simulink model "model2_sim"  (R2016a)
settings: Solver=VariableStepAuto  StartTime=0.0  StopTime=30  MaxStep=0.001  RelTol=1e-6
values from neighbouring files (symbols this model uses):
  damp_spring = 0    [model2.m]
  DC_delay = 0.005    [model1.m]    (also in model2.m)
  DC_max_force = 400    [model1.m]    (also in model2.m = 200)
  DC_PID_D = 0    [model1.m]    (also in model2.m = 1000)
  DC_PID_I = 0    [model1.m]    (also in model2.m)
  DC_PID_N = 100    [model2.m]
  DC_PID_P = 0    [model1.m]    (also in model2.m)
  k_cutoffspring = 20000    [model2.m]
  k_spring = 2500    [model2.m]
  linear_act_delay = 0.1    [model1.m]    (also in model2.m)
  linear_act_max = 0.25    [model1.m]    (also in model2.m = 0.5)
  linear_act_speed = 0.1    [model1.m]    (also in model2.m = 0.05)
  m_bed = 10    [model1.m]    (also in model2.m)
  m_payload = m_bed + m_patient    (= 40)    [model1.m]    (also in model2.m)
  max_offset = 0.1    [model1.m]    (also in model2.m)
  noise_rate = 0.1    [model1.m]    (also in model2.m)
  noise_rate_limit = 10    [model2.m]
  noise_start_time = 3    [model1.m]    (also in model2.m)
  patient_sit_pace = 50    [model2.m]
libraries: simulink x5, vrlib x3
settings Model: Creator=Perttu  LastModifiedBy=Perttu
settings SolverCC: InitialStep=0.0005

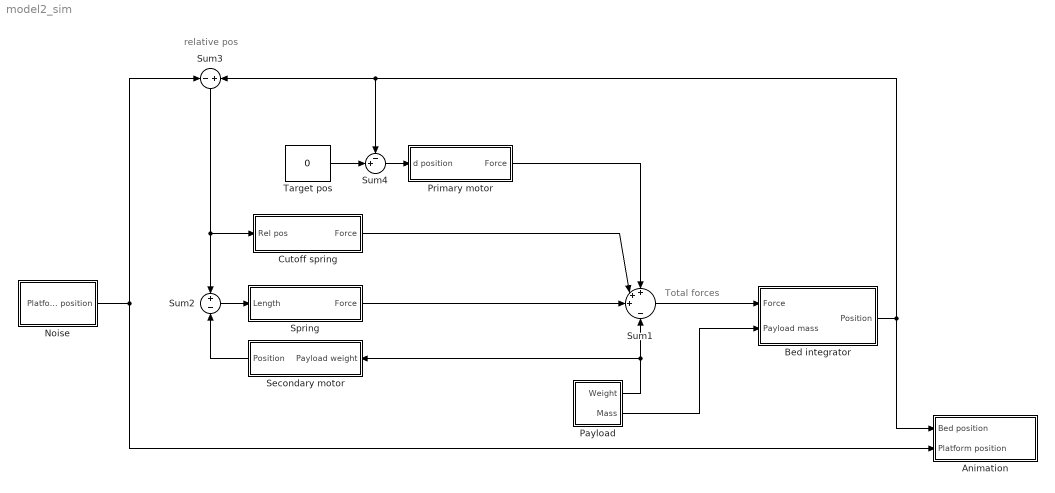
== system model2_sim ==
  note: relative pos
  note: Total forces
  Animation : Subsystem
  Bed integrator : Subsystem
  Cutoff spring : Subsystem
  Noise : Subsystem
  Payload : Subsystem
  Primary motor : Subsystem
  Secondary motor : Subsystem
  Spring : Subsystem
  Sum1 : Sum  Inputs=+++|-
  Sum2 : Sum  Inputs=+|-
  Sum3 : Sum  Inputs=-+
  Sum4 : Sum  Inputs=-+|
  Target pos : Constant  Value=0
  wires:
  Primary motor/1(Force) -> Sum1/1
  Sum2/1 -> Spring/1(Length)
  Payload/1(Weight) -> Sum1/4, Secondary motor/1(Payload weight)
  Sum4/1 -> Primary motor/1(d position)
  Target pos/1 -> Sum4/2
  Noise/1(Platform position) -> Animation/2(Platform position), Sum3/1
  Secondary motor/1(Position) -> Sum2/2
  Spring/1(Force) -> Sum1/3
  Bed integrator/1(Position) -> Animation/1(Bed position), Sum3/2, Sum4/1
  Payload/2(Mass) -> Bed integrator/2(Payload mass)
  Sum1/1 -> Bed integrator/1(Force)
  Cutoff spring/1(Force) -> Sum1/2
  Sum3/1 -> Sum2/1, Cutoff spring/1(Rel pos)

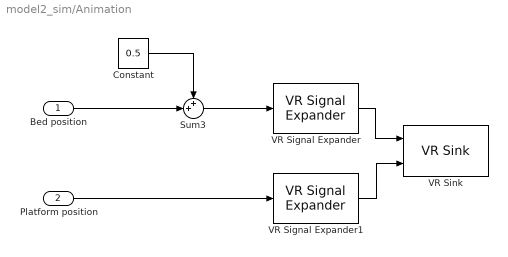
== system model2_sim/Animation ==
  Bed position : Inport
  Platform position : Inport  Port=2
  Constant : Constant  Value=0.5
  Sum3 : Sum  Inputs=++|
  VR Signal Expander : vrlib/VR Signal Expander  outwidth=3  outidx=[2]
  VR Signal Expander1 : vrlib/VR Signal Expander  outwidth=3  outidx=[2]
  VR Sink : vrlib/VR Sink  InstantiateOnLoad=on  SampleTime=0.03  ViewEnable=on  RemoteChange=off  RemoteView=off  FieldsWritten=Upper.translation.3.1.1.double#Lower.translation.3.1.1.double  WorldFileName=3dscene1.wrl  AutoView=on  VideoDimensions=[]  AllowVariableSize=off
  wires:
  Bed position/1 -> Sum3/2
  VR Signal Expander/1 -> VR Sink/1
  VR Signal Expander1/1 -> VR Sink/2
  Sum3/1 -> VR Signal Expander/1
  Constant/1 -> Sum3/1
  Platform position/1 -> VR Signal Expander1/1

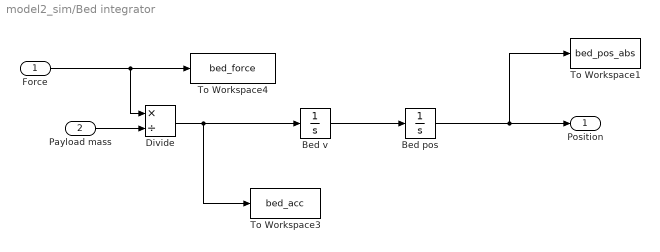
== system model2_sim/Bed integrator ==
  Force : Inport
  Payload mass : Inport  Port=2
  Bed pos : Integrator  UpperSaturationLimit=max_offset  LowerSaturationLimit=-max_offset  WrappedStateUpperValue=max_offset  WrappedStateLowerValue=-max_offset
  Bed v : Integrator
  Divide : Product  Inputs=*/
  To Workspace1 : ToWorkspace  VariableName=bed_pos_abs  SaveFormat=Timeseries  SampleTime=-1
  To Workspace3 : ToWorkspace  VariableName=bed_acc  SaveFormat=Timeseries  SampleTime=-1
  To Workspace4 : ToWorkspace  VariableName=bed_force  SaveFormat=Timeseries  SampleTime=-1
  Position : Outport
  wires:
  Force/1 -> To Workspace4/1, Divide/1
  Bed v/1 -> Bed pos/1
  Divide/1 -> To Workspace3/1, Bed v/1
  Payload mass/1 -> Divide/2
  Bed pos/1 -> To Workspace1/1, Position/1

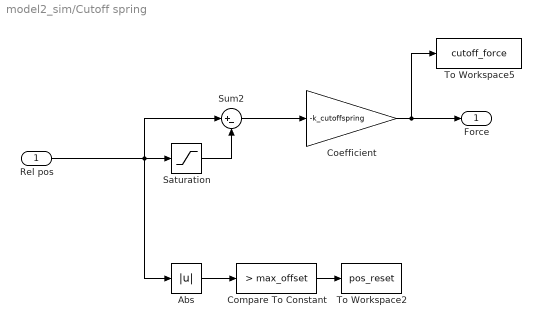
== system model2_sim/Cutoff spring ==
  Rel pos : Inport
  Abs : Abs
  Coefficient : Gain  Gain=-k_cutoffspring
  Compare To Constant : simulink/Logic and Bit Operations/Compare To Constant  relop=>  const=max_offset  OutDataTypeStr=boolean
  Saturation : Saturate  UpperLimit=max_offset  LowerLimit=-max_offset
  Sum2 : Sum  Inputs=|+-
  To Workspace2 : ToWorkspace  VariableName=pos_reset  SaveFormat=Timeseries  SampleTime=-1
  To Workspace5 : ToWorkspace  VariableName=cutoff_force  SaveFormat=Timeseries  SampleTime=-1
  Force : Outport
  wires:
  Compare To Constant/1 -> To Workspace2/1
  Rel pos/1 -> Abs/1, Saturation/1, Sum2/1
  Abs/1 -> Compare To Constant/1
  Saturation/1 -> Sum2/2
  Sum2/1 -> Coefficient/1
  Coefficient/1 -> Force/1, To Workspace5/1

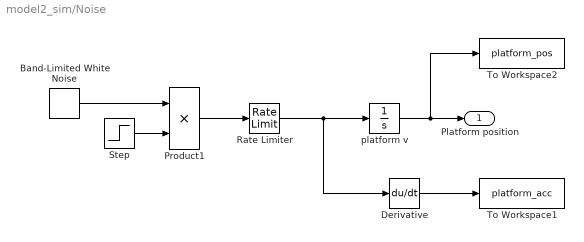
== system model2_sim/Noise ==
  Band-Limited White Noise : simulink/Sources/Band-Limited White Noise  Cov=noise_power  Ts=noise_rate  seed=noise_seed
  Derivative : Derivative
  Product1 : Product  OutDataTypeStr=Inherit: Same as first input
  Rate Limiter : RateLimiter  RisingSlewLimit=noise_rate_limit  FallingSlewLimit=-noise_rate_limit
  Step : Step  Time=noise_start_time  SampleTime=0
  To Workspace1 : ToWorkspace  VariableName=platform_acc  SaveFormat=Timeseries  SampleTime=-1
  To Workspace2 : ToWorkspace  VariableName=platform_pos  SaveFormat=Timeseries  SampleTime=-1
  platform v : Integrator
  Platform position : Outport
  wires:
  Band-Limited White Noise/1 -> Product1/1
  Step/1 -> Product1/2
  Product1/1 -> Rate Limiter/1
  platform v/1 -> To Workspace2/1, Platform position/1
  Derivative/1 -> To Workspace1/1
  Rate Limiter/1 -> Derivative/1, platform v/1

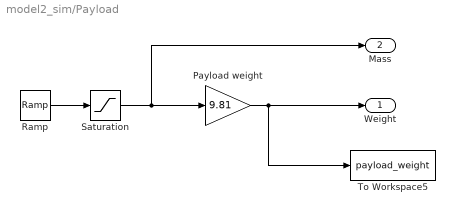
== system model2_sim/Payload ==
  Payload weight : Gain  Gain=9.81
  Ramp : simulink/Sources/Ramp  slope=patient_sit_pace  start=patient_sit_time  X0=m_bed
  Saturation : Saturate  UpperLimit=m_payload  LowerLimit=0
  To Workspace5 : ToWorkspace  VariableName=payload_weight  SaveFormat=Timeseries  SampleTime=-1
  Weight : Outport
  Mass : Outport  Port=2
  wires:
  Payload weight/1 -> To Workspace5/1, Weight/1
  Saturation/1 -> Mass/1, Payload weight/1
  Ramp/1 -> Saturation/1

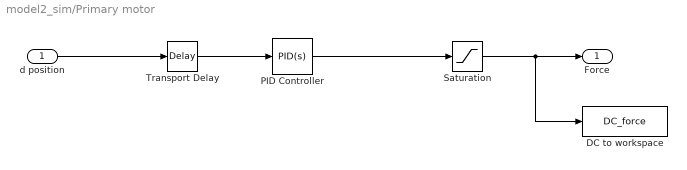
== system model2_sim/Primary motor ==
  d position : Inport
  DC to workspace : ToWorkspace  VariableName=DC_force  SaveFormat=Timeseries  SampleTime=-1
  PID Controller : simulink/Continuous/PID Controller  Controller=PID  TimeDomain=Continuous-time  SampleTime=-1  IntegratorMethod=Forward Euler  FilterMethod=Forward Euler  Form=Parallel  UseFilter=on  ControllerParametersSource=internal  P=DC_PID_P  I=DC_PID_I  D=DC_PID_D  N=DC_PID_N  InitialConditionSource=internal  InitialConditionForIntegrator=0  InitialConditionForFilter=0  ExternalReset=none  LimitOutput=off  UpperSaturationLimit=inf  LowerSaturationLimit=-inf  LinearizeAsGain=on  AntiWindupMode=none  Kb=1  TrackingMode=off  Kt=1  PParamMin=[]  PParamMax=[]  IParamMin=[]  IParamMax=[]  DParamMin=[]  DParamMax=[]  NParamMin=[]  NParamMax=[]  KbParamMin=[]  KbParamMax=[]  KtParamMin=[]  KtParamMax=[]  POutMin=[]  POutMax=[]  IOutMin=[]  IOutMax=[]  DOutMin=[]  DOutMax=[]  NOutMin=[]  NOutMax=[]  KbOutMin=[]  KbOutMax=[]  KtOutMin=[]  KtOutMax=[]  IntegratorOutMin=[]  IntegratorOutMax=[]  FilterOutMin=[]  FilterOutMax=[]  SumOutMin=[]  SumOutMax=[]  SumI1OutMin=[]  SumI1OutMax=[]  SumI2OutMin=[]  SumI2OutMax=[]  SumI3OutMin=[]  SumI3OutMax=[]  SumDOutMin=[]  SumDOutMax=[]  SaturationOutMin=[]  SaturationOutMax=[]  IntegratorContinuousStateAttributes=''  IntegratorStateMustResolveToSignalObject=off  IntegratorRTWStateStorageClass=Auto  FilterContinuousStateAttributes=''  FilterStateMustResolveToSignalObject=off  FilterRTWStateStorageClass=Auto  DifferentiatorICPrevScaledInput=0  DifferentiatorOutMin=[]  DifferentiatorOutMax=[]
  Saturation : Saturate  UpperLimit=DC_max_force  LowerLimit=-DC_max_force
  Transport Delay : TransportDelay  DelayTime=DC_delay  BufferSize=4096
  Force : Outport
  wires:
  Saturation/1 -> DC to workspace/1, Force/1
  PID Controller/1 -> Saturation/1
  d position/1 -> Transport Delay/1
  Transport Delay/1 -> PID Controller/1

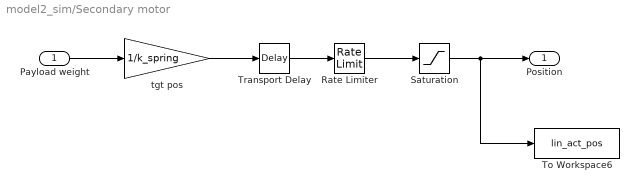
== system model2_sim/Secondary motor ==
  Payload weight : Inport
  Rate Limiter : RateLimiter  RisingSlewLimit=linear_act_speed  FallingSlewLimit=-linear_act_speed  SampleTimeMode=inherited  InitialCondition=m_bed * 9.81 / k_spring
  Saturation : Saturate  UpperLimit=linear_act_max  LowerLimit=0
  To Workspace6 : ToWorkspace  VariableName=lin_act_pos  SaveFormat=Timeseries  SampleTime=-1
  Transport Delay : TransportDelay  DelayTime=linear_act_delay  InitialOutput=m_bed * 9.81 / k_spring  BufferSize=4096
  tgt pos : Gain  Gain=1/k_spring
  Position : Outport
  wires:
  Payload weight/1 -> tgt pos/1
  Rate Limiter/1 -> Saturation/1
  Saturation/1 -> To Workspace6/1, Position/1
  Transport Delay/1 -> Rate Limiter/1
  tgt pos/1 -> Transport Delay/1

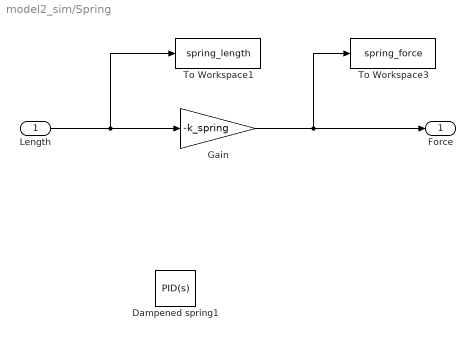
== system model2_sim/Spring ==
  Length : Inport
  Dampened spring1 : simulink/Continuous/PID Controller  Controller=PID  TimeDomain=Continuous-time  SampleTime=-1  IntegratorMethod=Forward Euler  FilterMethod=Forward Euler  Form=Parallel  UseFilter=on  ControllerParametersSource=internal  P=-k_spring  I=0  D=-damp_spring  N=100  InitialConditionSource=internal  InitialConditionForIntegrator=0  InitialConditionForFilter=0  ExternalReset=none  LimitOutput=off  UpperSaturationLimit=inf  LowerSaturationLimit=-inf  LinearizeAsGain=on  AntiWindupMode=none  Kb=1  TrackingMode=off  Kt=1  PParamMin=[]  PParamMax=[]  IParamMin=[]  IParamMax=[]  DParamMin=[]  DParamMax=[]  NParamMin=[]  NParamMax=[]  KbParamMin=[]  KbParamMax=[]  KtParamMin=[]  KtParamMax=[]  POutMin=[]  POutMax=[]  IOutMin=[]  IOutMax=[]  DOutMin=[]  DOutMax=[]  NOutMin=[]  NOutMax=[]  KbOutMin=[]  KbOutMax=[]  KtOutMin=[]  KtOutMax=[]  IntegratorOutMin=[]  IntegratorOutMax=[]  FilterOutMin=[]  FilterOutMax=[]  SumOutMin=[]  SumOutMax=[]  SumI1OutMin=[]  SumI1OutMax=[]  SumI2OutMin=[]  SumI2OutMax=[]  SumI3OutMin=[]  SumI3OutMax=[]  SumDOutMin=[]  SumDOutMax=[]  SaturationOutMin=[]  SaturationOutMax=[]  IntegratorContinuousStateAttributes=''  IntegratorStateMustResolveToSignalObject=off  IntegratorRTWStateStorageClass=Auto  FilterContinuousStateAttributes=''  FilterStateMustResolveToSignalObject=off  FilterRTWStateStorageClass=Auto  DifferentiatorICPrevScaledInput=0  DifferentiatorOutMin=[]  DifferentiatorOutMax=[]
  Gain : Gain  Gain=-k_spring
  To Workspace1 : ToWorkspace  VariableName=spring_length  SaveFormat=Timeseries  SampleTime=-1
  To Workspace3 : ToWorkspace  VariableName=spring_force  SaveFormat=Timeseries  SampleTime=-1
  Force : Outport
  wires:
  Gain/1 -> Force/1, To Workspace3/1
  Length/1 -> Gain/1, To Workspace1/1
